simulink model "andGatter"  (R2018b)
settings: Solver=VariableStepAuto  StartTime=0.0  StopTime=10.0  RelTol=1e-3
settings Model: Creator=ms  LastModifiedBy=ms

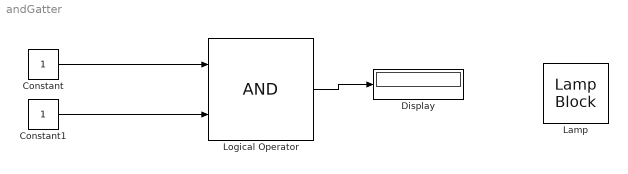
== system andGatter ==
  Constant : Constant
  Constant1 : Constant
  Display : Display
  Lamp : LampBlock  WebBlockId=16
  Logical Operator : Logic  AllPortsSameDT=off  OutDataTypeStr=boolean
  wires:
  Constant/1 -> Logical Operator/1
  Constant1/1 -> Logical Operator/2
  Logical Operator/1 -> Display/1
